simulink model "cart_pend_AMPC_with_DMDc"  (R2019b)
settings: Solver=FixedStepAuto  StartTime=0.0  StopTime=50  FixedStep=0.01  RelTol=1e-3
values from neighbouring files (symbols this model uses):
  A = [0.969169519504925  -0.246386829627017;  0.049277365925403  0.993808202467626]    [DMDc_MW.m]    (also in DMDc_param_sweep.m = real(A); EKF_msd_estimator.m = [0, 1; -k/m, -b/m]; HAVOK.m = AB(:,1:q*m); HAVOK_param_sweep.m = real(A))
  B = [0.049277365925403; 0.001238359506475]    [DMDc_MW.m]    (also in DMDc_param_sweep.m = AB(:,(q*m+1):end); EKF_estimator.m = zeros(nx,1); EKF_msd_estimator.m = [0; 1/m]; HAVOK.m = AB(:,(q*m+1):end))
  C = [0 1]    [DMDc_MW.m]    (also in EKF_estimator.m = eye(6); EKF_msd_estimator.m = [1, 0]; KF_estimator.m = [1, 0]; LS.m)
  D = 0    [DMDc_MW.m]    (also in DMDc_param_sweep.m = (q-1)*Ts; EKF_estimator.m = m*L*L*(M+m*(1-Cx^2)); EKF_msd_estimator.m; HAVOK.m = 3.99)
  DX = [0; 0]    [DMDc_MW.m]    (also in LS.m; cart_pend_DMD_script.m; convert_model_for_AMPC.m; mass_spring_damper_DMD_script.m)
  nu = size_B(2)    [DMDc_MW.m]    (also in EKF_msd_estimator.m = 1; LS.m; Linear_regression_state_estimator.m = 2; cart_pend_DMD_script.m)
  ny = size_C(1)    [DMDc_MW.m]    (also in EKF_msd_estimator.m = 1; LS.m; Linear_regression_state_estimator.m = 1; cart_pend_DMD_script.m)
  p = 200    [HAVOK.m]    (also in cart_pend_HAVOK_N_train_time_sweep.m = p_saved(index); cart_pend_HAVOK_script.m = 40; floating_pend_2D_HAVOK_script.m = p_saved(save_index); mass_spring_damper_DMD_script.m = size(V)*[0; 1])
  Ts = 0.05    [DMDc_MW.m]    (also in DMDc_param_sweep.m = t(2)-t(1); EKF_msd_estimator.m = 0.01; HAVOK.m = t(2)-t(1); HAVOK_param_sweep.m = t(2)-t(1))
  U = zeros(nu,1)    [DMDc_MW.m]    (also in HAVOK.m = u_train(:, q:end-1); LS.m; Linear_regression_state_estimator.m = reshape(U, nx*nu,1); cart_pend_DMD_script.m)
  X = zeros(nx,1)    [DMDc_MW.m]    (also in LS.m; Linear_regression_parameter_estimator.m = [y_data(2:end-1)', y_data(1:end-2)', u_data(1:end-2)']; cart_pend_DMD_script.m; cart_pend_HAVOK_N_train_error_sweep.m = zeros(q*m,w))
  Y = zeros(ny,1)    [DMDc_MW.m]    (also in DMDc_param_sweep.m = zeros(q*m,w); HAVOK.m = zeros(q*m,w); HAVOK_param_sweep.m = zeros(q*m,w); LS.m)
undefined symbols (not defined in the file or in its folder): blk, iA, isLTV, lastPcov, lastu, lastx, MDscale, MVscale, nCC, nud, nv, nxp, nym, RMVscale, RYscale, ts, uoff, xoff, Yscale
libraries: mpcsigdimcheck_private x23, mpclib x1
(part 2 of 2)

== matlab function cart_pend_AMPC_with_DMDc/Adaptive MPC Controller/MPC/optimizer/VariableHorizonOptimizer ==
  settings: updateMethod=DISCRETE  sampleTime=ts
  data: xk1 output BlockDataType; xk input BlockDataType; old_u input BlockDataType; ym input BlockDataType; ref input BlockDataType; md input BlockDataType; umin input BlockDataType; umax input BlockDataType; ymin input BlockDataType; ymax input BlockDataType; E input BlockDataType; F input BlockDataType; G input BlockDataType; S input BlockDataType; switch_in input BlockDataType; ext_mv input BlockDataType; MVtarget input BlockDataType; isQP parameter boolean; nx parameter BlockDataType; nxp parameter BlockDataType; nup parameter BlockDataType; nu parameter BlockDataType; ny parameter BlockDataType; degrees parameter BlockDataType; Mlim parameter BlockDataType; Mx parameter BlockDataType; Mu1 parameter BlockDataType; Mv parameter BlockDataType; utarget parameter BlockDataType; p parameter BlockDataType; maxiter parameter BlockDataType; CustomSolver parameter boolean; CustomSolverCodeGen parameter boolean; UseSuboptimalSolution parameter boolean; nxQP parameter BlockDataType; openloopflag parameter boolean; no_umin parameter BlockDataType; no_umax parameter BlockDataType; no_ymin parameter BlockDataType; no_ymax parameter BlockDataType; switch_inport parameter BlockDataType; no_switch parameter BlockDataType; enable_value parameter BlockDataType; return_cost parameter BlockDataType; H parameter BlockDataType; return_mvseq parameter BlockDataType; return_xseq parameter BlockDataType; return_ovseq parameter BlockDataType; Ac parameter BlockDataType; ywt input BlockDataType; uwt input BlockDataType; duwt input BlockDataType; rhoeps input BlockDataType; isLTV parameter boolean; a input BlockDataType; b input BlockDataType; c input BlockDataType; d input BlockDataType; U input BlockDataType; Y input BlockDataType; X input BlockDataType; DX input BlockDataType; Pk input BlockDataType; iA input boolean; extp input BlockDataType; extm input BlockDataType; u output BlockDataType; cost output BlockDataType; useq output BlockDataType; xseq output BlockDataType; yseq output BlockDataType; status output BlockDataType; xest output BlockDataType; Pk1 output BlockDataType; no_ywt parameter BlockDataType; no_uwt parameter BlockDataType; no_duwt parameter BlockDataType; no_rhoeps parameter BlockDataType; Wy parameter BlockDataType; Wdu parameter BlockDataType; Wu parameter BlockDataType; iAout output boolean; A parameter BlockDataType; C parameter BlockDataType; B parameter BlockDataType; D parameter BlockDataType; Cid parameter BlockDataType; Did parameter BlockDataType; Mrows parameter BlockDataType; nCC parameter BlockDataType; Ecc parameter BlockDataType; Fcc parameter BlockDataType; Scc parameter BlockDataType; Gcc parameter BlockDataType; nv parameter BlockDataType; no_md parameter BlockDataType; no_ref parameter BlockDataType; no_uref parameter BlockDataType; no_mv parameter BlockDataType; RYscale parameter BlockDataType; RMDscale parameter BlockDataType; myindex parameter BlockDataType; xoff parameter BlockDataType; CustomEstimation parameter boolean; mvindex parameter BlockDataType; mdindex parameter BlockDataType; unindex parameter BlockDataType; nxid parameter BlockDataType; Uscale parameter BlockDataType; Yscale parameter BlockDataType; uoff parameter BlockDataType; voff parameter BlockDataType; yoff parameter BlockDataType; myoff parameter BlockDataType; no_cc parameter BlockDataType; p0 parameter
function [xk1, u, cost, useq, xseq, yseq, status, xest, Pk1, iAout] = fcn(...
            xk, old_u, ym, ref, md, umin, umax, ymin, ymax, E, F, G, S,...
            switch_in, ext_mv, MVtarget, isQP, nx, nxp, nup, ...
            nu, ny, degrees, Mlim, ...
            Mx, Mu1, Mv, utarget, p, maxiter, ...
            CustomSolver, CustomSolverCodeGen, UseSuboptimalSolution, nxQP, openloopflag, ...
            no_umin, no_umax, no_ymin, no_ymax, switch_inport, no_switch, enable_value, ...
            return_cost, H, return_mvseq, return_xseq, return_ovseq, Ac, ...
            ywt, uwt, duwt, rhoeps, isLTV, a, b, c, d, U, Y, X, DX, Pk, iA, extp, extm, ...
            no_ywt, no_uwt, no_duwt, no_rhoeps,...
            Wy, Wdu, Wu, A, C, B, D, Cid, Did, Mrows, nCC, Ecc, Fcc, Scc, Gcc, ...
            nv, no_md, no_ref, no_uref, no_mv, RYscale, RMDscale, myindex, ...
            xoff, CustomEstimation, mvindex, mdindex, unindex, nxid, Uscale, Yscale, uoff, voff, yoff, myoff, no_cc, ...
            p0)
%#codegen
coder.extrinsic('mpcblock_optimizerPM_double_mex');
coder.extrinsic('mpcblock_optimizerPM_single_mex');
coder.extrinsic('mpcblock_refmd_double_mex');
coder.extrinsic('mpcblock_refmd_single_mex');

% The following is for DEBUG:
%%%%%%%%%%%%%%%
% coder.extrinsic('mpcblock_optimizerPM');
%%%%%%%%%%%%%%%

% Constants
isSimulation = coder.target('Sfun') && ~coder.target('RtwForRapid') && ~coder.target('RtwForSim');
isAdaptive = ~isLTV; % isLTV=true forces isAdaptive=false
isDouble = isa(ref,'double');
if isDouble
    DataType = 'double';
else
    DataType = 'single';
end
ZERO = zeros('like',ref);
ONE = ones('like',ref);
hasMD = nv>1;

% Keep output arguments related to prediction horizon (useq,xseq,yseq) of 
% size pmax, so that they don't change dimension in case extp varies. 
% Here pmax = input parameter 'p'.

% Pre-allocate all the MEX block outputs for the simulation mode
%#ok<*NASGU>
if isSimulation
    rseq = zeros(extp*ny,1,'like',ref); %#ok<*NASGU>
    vseq = zeros((extp+1)*nv,1,'like',ref);
    v = zeros(nv,1,'like',ref);
    xk1 = zeros(nx,1,'like',ref);
    u = zeros(nu,1,'like',ref);
    cost = ZERO;
    useq = zeros(p+1,nu,'like',ref); %#ok<*PREALL>
    status = ONE;
    xest = zeros(nx,1,'like',ref);
    iAout = iA;
end

% Model update
nym = length(myindex);
ai=zeros(nxp,nxp,'like',ref);
bi=zeros(nxp,nup,'like',ref);
ci=zeros(ny,nxp,'like',ref);
di=zeros(ny,nup,'like',ref);

ai(:,:)=a(:,:,1);
bi(:,:)=b(:,:,1);
ci(:,:)=c(:,:,1);
di(:,:)=d(:,:,1);

% Allocate matrices. Must allocate 3D matrix also in Adaptive case,
% otherwise EML code does not compile.
Bu=zeros(nx,nu,extp+1,'like',ref);
Bv=zeros(nx,nv,extp+1,'like',ref);
Dv=zeros(ny,nv,extp+1,'like',ref);
Dvm=zeros(nym,nv,extp+1,'like',ref);
Cm=zeros(nym,nx,extp+1,'like',ref);
if ~isLTV
    % Adaptive
    [A(:,:,1),C(:,:,1),Bu(:,:,1),Bv(:,:,1),Cm(:,:,1),Dv(:,:,1),Dvm(:,:,1),Qk,Rk,Nk] = mpc_plantupdate(...
        ai,bi,ci,di,A(:,:,1),B(:,:,1),C(:,:,1),D(:,:,1),mvindex,mdindex,unindex,nxp,nup,ny,nv,nxid, ...
        myindex,Uscale,Yscale,Cid,Did);
else
    % Retrieve LTV model
    for i=1:extp+1
        ai(1:nxp,1:nxp)=a(:,:,i);
        bi(1:nxp,1:nup)=b(:,:,i);
        ci(1:ny,1:nxp)=c(:,:,i);
        di(1:ny,1:nup)=d(:,:,i);
        [A(:,:,i),C(:,:,i),Bu(:,:,i),Bv(:,:,i),Cm(:,:,i),Dv(:,:,i),Dvm(:,:,i),Qk,Rk,Nk] =...
            mpc_plantupdate(ai,bi,ci,di,A(:,:,i),B(:,:,i),C(:,:,i),D(:,:,i),mvindex,mdindex,unindex,nxp,nup,ny,nv,nxid, ...
            myindex,Uscale,Yscale,Cid,Did);
    end
end

% Offset update together with Mlim, utarget, Bv and Dv values
[Mlim, utarget, uoff, voff, yoff, myoff, xoff, Bv, Dv] = ...
    mpc_updateFromNominal(isAdaptive,isQP,p0,Mlim,Mrows,...
       U,Uscale,uoff,mvindex,voff,mdindex,utarget,nu,nv-1,...
       Y,Yscale,yoff,myoff,myindex,ny,...
       X,xoff,nxp,DX,A,Bu,Bv,C,Dv,nCC);

% Remove last u offset
old_u = old_u - uoff;       

% Get reference and MD signals -- accounting for previewing
if isSimulation
    if isDouble
        %%%%%%%%%%%%%%%%%%%%%%%%%%%%%%%%%%%%%%%%%%%%%
        %%%%%% TEMPORARILY DISABLE MEX FILE %%%%%%%%%
        %%%%%%%%%%%%%%%%%%%%%%%%%%%%%%%%%%%%%%%%%%%%%
        [rseq, vseq, v] = mpcblock_refmd_double_mex(ref,md,nv,ny,extp,yoff,voff,no_md,no_ref,openloopflag, RYscale, RMDscale);
        %[rseq, vseq, v] = mpcblock_refmd(ref,md,nv,ny,extp,yoff,voff,no_md,no_ref,openloopflag, RYscale, RMDscale);
    else
        %%%%%%%%%%%%%%%%%%%%%%%%%%%%%%%%%%%%%%%%%%%%%
        %%%%%% TEMPORARILY DISABLE MEX FILE %%%%%%%%%
        %%%%%%%%%%%%%%%%%%%%%%%%%%%%%%%%%%%%%%%%%%%%%
        [rseq, vseq, v] = mpcblock_refmd_single_mex(ref,md,nv,ny,extp,yoff,voff,no_md,no_ref,openloopflag, RYscale, RMDscale);        
        %[rseq, vseq, v] = mpcblock_refmd(ref,md,nv,ny,extp,yoff,voff,no_md,no_ref,openloopflag, RYscale, RMDscale);        
    end
else
    % When doing code generation, use M code directly
    [rseq, vseq, v] = mpcblock_refmd(ref,md,nv,ny,extp,yoff,voff,no_md,no_ref,openloopflag, RYscale, RMDscale);
end

% External MV override.  
% NOTE: old_u and ext_mv input signals are dimensionless and offset-free.
if no_mv==ONE
    % no external mv: old_u is the optimal u[k-1] from last_mv
    delmv = zeros(nu,1,'like',ref);
else
    % has external mv: old_u is the external u[k-1]
    ext_mv = ext_mv - uoff;     % bias correction
    delmv = ext_mv - old_u;
    old_u = ext_mv;
end

% Obtain x[k|k]
xk = xk - xoff;     % Remove offset
if CustomEstimation==ONE
    % Input is x(k|k)
    xest = xk;
else
    % Calculate gain matrices, and perform measurement update.
    Kinv = eye(nym,'like',ref)/(Cm(:,:,1)*Pk*Cm(:,:,1)' + Rk);
    L = (A(:,:,1)*Pk*Cm(:,:,1)' + Nk)*Kinv;
    M = Pk*Cm(:,:,1)'*Kinv;
    % LTVKF state estimation.
    % Scale measured output and remove offset.
    ym = ym.*RYscale(myindex) - myoff;
    % Correct x(k|k-1) for possible external mv override.
    % NOTE:  Offset was removed from x[k|k-1] at k=0.
    xk = xk + Bu(:,:,1)*delmv;
    % Measurement upate to x(k|k)
    ym_est = Cm(:,:,1)*xk + Dvm(:,:,1)*v;
    y_innov = ym - ym_est;
    xest = xk + M*y_innov;
end

% Real-time MV target override
% Note: utargetValue is a vector length p*nu.  
if no_uref==ONE
    % no external utarget
    utargetValue = utarget;
else
    % Define constant targets for the entire horizon.
    MVtarget = MVtarget - uoff;         % Bias correction
    utargetValue = reshape(MVtarget(:,ones(p,1)),nu*p,1);
end

% Real-time custom constraint override (scaled E/F/S)
if no_cc~=ONE
    Ecc = E;
    Fcc = F;
    Gcc = G;
    if nv>1
        Scc = S;
    end
end

return_sequence = (return_mvseq || return_xseq || return_ovseq)*ONE;

if numel(extm) > 1
    nMoves = numel(extm)*nu;
    %extm(end) = extp - sum(extm(1:end-1));
else
    nMoves = extm*nu;
    %extm = [ones(1,extm-1), extp-extm+1];
end
extdegrees=nMoves+isQP;
extz_degrees = zeros(extdegrees,1,'like',ref);

% The following is for DEBUG:
%%%%%%%%%%%%%%%
% u=zeros(nu,1,'like',ref);
% cost=ZERO;
% useq1=zeros(p+1,nu,'like',ref);
% status=ZERO;
% iAout=false(size(iA));
%%%%%%%%%%%%%%%

if isSimulation
    if isDouble
        %%%%%%%%%%%%%%%%%%%%%%%%%%%%%%%%%%%%%%%%%%%%%
        %%%%%% TEMPORARILY DISABLE MEX FILE %%%%%%%%%
        %%%%%%%%%%%%%%%%%%%%%%%%%%%%%%%%%%%%%%%%%%%%%
        %[u, cost, useq1, status, iAout] = mpcblock_optimizerPM(...
        [u, cost, useq1, status, iAout] = mpcblock_optimizerPM_double_mex(...
            rseq, vseq, umin, umax, ymin, ymax, switch_in, xest, old_u, iA, isQP, nu, ny, ...
            Mlim, Mx, Mu1, Mv, extz_degrees, ...
            utargetValue, extp, extm, uoff, voff, yoff, maxiter,...
            CustomSolver, false, UseSuboptimalSolution, nxQP, openloopflag,...
            no_umin, no_umax, no_ymin, no_ymax, switch_inport,...
            no_switch, enable_value, return_cost, H, return_sequence, Ac,...
            ywt, uwt, duwt, rhoeps, no_ywt, no_uwt, no_duwt, no_rhoeps,...
            Wy, Wdu, Wu, isLTV, A, Bu, Bv, C, Dv,...
            Mrows, nCC, Ecc, Fcc, Scc, Gcc,...
            p0,degrees,p);    
    else
        %%%%%%%%%%%%%%%%%%%%%%%%%%%%%%%%%%%%%%%%%%%%%
        %%%%%% TEMPORARILY DISABLE MEX FILE %%%%%%%%%
        %%%%%%%%%%%%%%%%%%%%%%%%%%%%%%%%%%%%%%%%%%%%%
        %[u, cost, useq1, status, iAout] = mpcblock_optimizerPM(...
        [u, cost, useq1, status, iAout] = mpcblock_optimizerPM_single_mex(...
            rseq, vseq, umin, umax, ymin, ymax, switch_in, xest, old_u, iA, ...
            isQP, nu, ny, Mlim, ...
            Mx, Mu1, Mv, extz_degrees, utargetValue, extp, extm, uoff, voff, yoff, maxiter, ...
            CustomSolver, false, UseSuboptimalSolution, nxQP, openloopflag, ...
            no_umin, no_umax, no_ymin, no_ymax, switch_inport, ...
            no_switch, enable_value, return_cost, H, return_sequence, Ac, ...
            ywt, uwt, duwt, rhoeps, no_ywt, no_uwt, no_duwt, no_rhoeps,...
            Wy, Wdu, Wu, isLTV, A, Bu, Bv, C, Dv, ...
            Mrows, nCC, Ecc, Fcc, Scc, Gcc, ...
            p0,degrees,p);    
    end
else
    % When doing code generation, use M code directly
        [u, cost, useq1, status, iAout] = mpcblock_optimizerPM(...
            rseq, vseq, umin, umax, ymin, ymax, switch_in, xest, old_u, iA, ...
            isQP, nu, ny, Mlim, ...
            Mx, Mu1, Mv, extz_degrees, utargetValue, extp, extm, uoff, voff, yoff, maxiter, ...
            false, CustomSolverCodeGen, UseSuboptimalSolution, nxQP, openloopflag, ...
            no_umin, no_umax, no_ymin, no_ymax, switch_inport, ...
            no_switch, enable_value, return_cost, H, return_sequence, Ac, ...
            ywt, uwt, duwt, rhoeps, no_ywt, no_uwt, no_duwt, no_rhoeps,...
            Wy, Wdu, Wu, isLTV, A, Bu, Bv, C, Dv, ...
            Mrows, nCC, Ecc, Fcc, Scc, Gcc, ...
            p0,degrees,p);
end

% Add missing zeros in useq
useq = zeros(p+1,nu,'like',rseq);
for k=1:p+1
    if k<=extp+1
        for i=1:nu
            useq(k,i)=useq1(k,i);
        end
    end
end

if return_xseq || return_ovseq
    [yseq, xseq] = mpc_computeSequence(isLTV, xest, useq, vseq, uoff, yoff, xoff, extp, ny, nxQP, nv, A, Bu, Bv, C, Dv);
else
    yseq = zeros(p+1,ny,'like',rseq);
    xseq = zeros(p+1,nxQP,'like',rseq);
end

if CustomEstimation==ONE
    xk1 = zeros(nx,1,'like',ref);
    Pk1 = Pk;
else
    % LTVKF state and covariance update
    xk1 = A(:,:,1)*xk + Bu(:,:,1)*(u - uoff) + Bv(:,:,1)*v + L*y_innov;
    Pk1 = A(:,:,1)*Pk*A(:,:,1)' - (A(:,:,1)*Pk*Cm(:,:,1)' + Nk)*L' + Qk;
    Pk1 = 0.5*(Pk1 + Pk1'); % guarantee symmetric for numerical stability
end
xk1 = xk1 + xoff;   % Updated state must include offset

% return xest in original value
xest = xest + xoff;
